simulink model "s9_template"  (R2023b)
settings: Solver=ode4  StartTime=0.0  StopTime=inf  FixedStep=P_sim_dt  RelTol=1e-3
InitFcn:
  | %madctrl_data;
  | s6_data;
values from neighbouring files (symbols this model uses):
  a1total = 2.70    (= 2.7)    [s6_data.m]
  a2total = 1.8    [s6_data.m]
  CarInputsCmdForward = uint8(1)    [p_mad_car.m]
  CarInputsCmdHalt = uint8(0)    [p_mad_car.m]
  CarInputsCmdReverse = uint8(2)    [p_mad_car.m]
  CarInputsCmdSlow = uint8(3)    [p_mad_car.m]
  P_k_p = 1    [s6_data.m]
  P_kr = 0.3440    (= 0.344)    [s6_data.m]
  P_ManeuverTypePark = 1    [s6_data.m]
  P_ManeuverTypePathFollow = 0    [s6_data.m]
  P_p_Bf = 0.7    [p_mad_car.m]
  P_p_Br = 0.7    [p_mad_car.m]
  P_p_Cf = 2    [p_mad_car.m]
  P_p_Cr = 2    [p_mad_car.m]
  P_p_delta_max = 21.58/180*pi    (= 0.37664205258)    [p_mad_car.m]
  P_p_Df = 2    [p_mad_car.m]
  P_p_Dr = 2.5    [p_mad_car.m]
  P_p_Ef = -0.1    [p_mad_car.m]
  P_p_Er = -0.05    [p_mad_car.m]
  P_p_J = 192e-6    (= 0.000192)    [p_mad_car.m]
  P_p_k = 2.51    [p_mad_car.m]
  P_p_l = abs(P_p_frontaxle_1 + P_p_rearaxle_1)    [p_mad_car.m]
  P_p_lf = P_p_frontaxle_1    (= 0.05)    [p_mad_car.m]
  P_p_lr = P_p_rearaxle_1    (= 0.049)    [p_mad_car.m]
  P_p_m = 132e-3    (= 0.132)    [p_mad_car.m]
  P_p_own = [P_p_s10; P_p_s20; 0; 0; 0; 0; 0 ]    [p_mad_car.m]
  P_p_T = 316e-3    (= 0.316)    [p_mad_car.m]
  P_p_Tt = P_p_uTt + P_p_output_Tt    (= 0.1)    [p_mad_car.m]
  P_p_Tw = 300e-3    (= 0.3)    [s6_data.m]
  P_prevent_buffer = 0.1    [s6_data.m]
  P_safety_buffer = 0.05    [s6_data.m]
  P_Ta = 20e-3    (= 0.02)    [s6_data.m]
  P_Ti = 0.2468    [s6_data.m]
  P_w_breakslen = uint32(length(path.points))    [s6_data.m]
  P_w_coefs = zeros(SPLINE.Elements(3).Dimensions)    [s6_data.m]
  P_w_points = zeros(SPLINE.Elements(2).Dimensions)    [s6_data.m]
  P_w_segments = uint32(zeros(SPLINE.Elements(4).Dimensions))    [s6_data.m]
  P_xManeuverEnd = 1    [s6_data.m]
  points = [p.x+x; s1; s2]    [mbc_clothoid_get_points.m]
undefined symbols (not defined in the file or in its folder): breakslen, coefs, DiscIntNeverNeededParam, periodic, segments
libraries: mad_lib_template x1, simulink x1
(part 2 of 2)

== matlab function s9_template/vehicle_dynamics/vehicle_dynamics_highspeed/calculate_beta ==
  data: v_c1 input; beta output; v_c2 input
function beta = calculate_beta(v_c1, v_c2)
    % Function: calculate_beta
    % Description: Calculates the sideslip angle 'beta' of a vehicle based on its
    %              longitudinal and lateral velocity components.
    %
    % Inputs:
    %   v_c1 [m/s] - Longitudinal velocity component of the vehicle.
    %   v_c2 [m/s] - Lateral velocity component of the vehicle.
    %
    % Output:
    %   beta [rad] - Calculated sideslip angle.
    %
    % The function uses the 'atan2' function for a more accurate calculation of the
    % angle, especially in cases where the longitudinal velocity component (v_c1) is zero.
    % The sideslip angle 'beta' is an important parameter in vehicle dynamics, representing
    % the angle between the vehicle's direction of motion and the direction it's pointing.
    %
    % Calculation of the sideslip angle 'beta'
    beta = atan2(v_c2, v_c1);
end

== matlab function s9_template/vehicle_dynamics/vehicle_dynamics_highspeed/calculate_s1_p_and_s2_p ==
  data: v_c1 input; s1_p output; v_c2 input; psi input; s2_p output
function [s1_p, s2_p] = calculate_s1_p_and_s2_p(v_c1, v_c2, psi)
    % Function: calculate_s1_p_and_s2_p
    % Description: Transforms the velocity components from the vehicle's coordinate
    %              system to the global coordinate system.
    %
    % Inputs:
    %   v_c1 [m/s] - Longitudinal velocity component in the vehicle's coordinate system.
    %   v_c2 [m/s] - Lateral velocity component in the vehicle's coordinate system.
    %   psi [rad] - Yaw angle of the vehicle.
    %
    % Outputs:
    %   s1_p [m/s] - Transformed longitudinal velocity component in the global coordinate system.
    %   s2_p [m/s] - Transformed lateral velocity component in the global coordinate system.
    %
    % The function applies a 2D rotation transformation to the velocity components (v_c1, v_c2)
    % based on the vehicle's yaw angle (psi). This transformation is useful for converting
    % vehicle-relative velocities to a global reference frame.

    % Calculating the transformed velocity components
    s1_p = v_c1 * cos(psi) - v_c2 * sin(psi);
    s2_p = v_c1 * sin(psi) + v_c2 * cos(psi);
end
